simulink model "Aeropendulum_test_simple"  (R2021b)
settings: Solver=VariableStepAuto  StartTime=0.0  StopTime=10.0  RelTol=1e-3
values from neighbouring files (symbols this model uses):
  c = 0.007    [ANM_params.m]    (also in ANM_params_test.m)
  d = 0.25    [ANM_params.m]    (also in ANM_params_test.m)
  g = 9.81    [ANM_params.m]    (also in ANM_params_test.m)
  J = m*l*l    (= 0.0075)    [ANM_params.m]    (also in ANM_params_test.m)
  l = 0.25    [ANM_params.m]    (also in ANM_params_test.m)
  m = 0.120    (= 0.12)    [ANM_params.m]    (also in ANM_params_test.m)
  Rs = 5    [ANM_params.m]
libraries: simulink x1
settings Model: Creator=Marcin  LastModifiedBy=Marcin

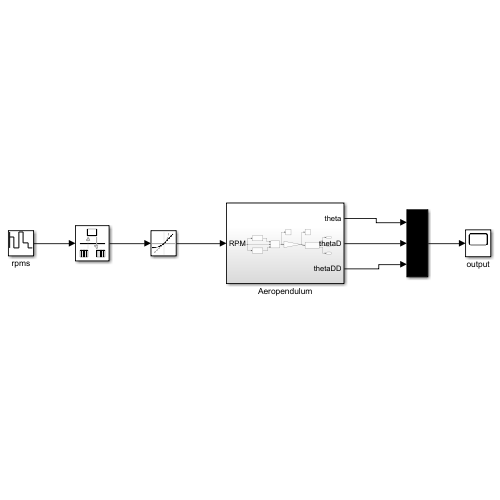
[thumbnail: Simulink's stored preview of the top-level diagram]
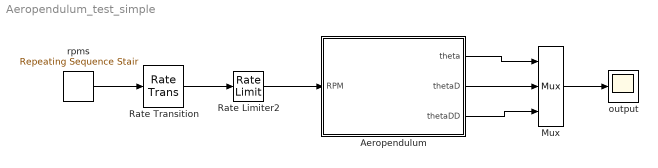
== system Aeropendulum_test_simple ==
  Aeropendulum : Subsystem
  Mux : Mux  Inputs=3
  Rate Limiter2 : RateLimiter  RisingSlewLimit=Rs  FallingSlewLimit=-Rs  SampleTimeMode=inherited
  Rate Transition : RateTransition  InitialCondition=10  OutPortSampleTime=Ts
  output : Scope
  rpms : simulink/Sources/Repeating Sequence Stair  OutValues=input_yref_vector  tsamp=Ts  OutMin=[]  OutMax=[]  OutDataTypeStr=double  OutputDataTypeScalingMode=double  OutDataType=fixdt(0,8)  ConRadixGroup=Best Precision: Vector-wise  OutScaling=2^-12
  wires:
  Rate Transition/1 -> Rate Limiter2/1
  rpms/1 -> Rate Transition/1
  Mux/1 -> output/1
  Aeropendulum/1(theta) -> Mux/1
  Aeropendulum/2(thetaD) -> Mux/2
  Aeropendulum/3(thetaDD) -> Mux/3
  Rate Limiter2/1 -> Aeropendulum/1(RPM)

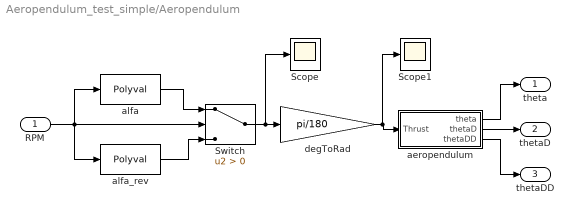
== system Aeropendulum_test_simple/Aeropendulum ==
  RPM : Inport
  Scope : Scope
  Scope1 : Scope
  Switch : Switch  Criteria=u2 > Threshold
  aeropendulum : Subsystem
  alfa : Polyval  Coefs="[3.04986021927422e-06,  -0.00476887717971010 , 2.51670431281220]"
  alfa_rev : Polyval  Coefs="[-5.46944010985214e-06,\t-0.00938361577873603,\t-2.43262552689868]"
  degToRad : Gain  Gain=pi/180
  theta : Outport
  thetaD : Outport  Port=2
  thetaDD : Outport  Port=3
  wires:
  alfa/1 -> Switch/1
  RPM/1 -> alfa_rev/1, alfa/1, Switch/2
  Switch/1 -> Scope/1, degToRad/1
  degToRad/1 -> Scope1/1, aeropendulum/1(Thrust)
  alfa_rev/1 -> Switch/3
  aeropendulum/1(theta) -> theta/1
  aeropendulum/2(thetaD) -> thetaD/1
  aeropendulum/3(thetaDD) -> thetaDD/1

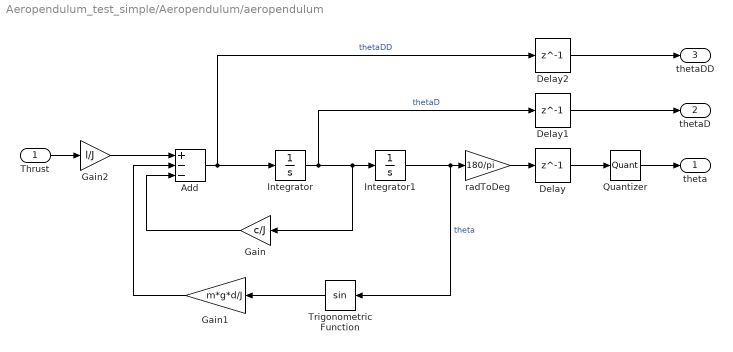
== system Aeropendulum_test_simple/Aeropendulum/aeropendulum ==
  Thrust : Inport
  Add : Sum  Inputs=+--
  Delay : Delay  DelayLength=1  InitialCondition=0
  Delay1 : Delay  DelayLength=1  InitialCondition=0
  Delay2 : Delay  DelayLength=1  InitialCondition=0
  Gain : Gain  Gain=c/J
  Gain1 : Gain  Gain=m*g*d/J
  Gain2 : Gain  Gain=l/J
  Integrator : Integrator
  Integrator1 : Integrator
  Quantizer : Quantizer  QuantizationInterval=0.08791209
  Trigonometric Function : Trigonometry
  radToDeg : Gain  Gain=180/pi
  theta : Outport
  thetaD : Outport  Port=2
  thetaDD : Outport  Port=3
  wires:
  Thrust/1 -> Gain2/1
  Integrator/1 -> Delay1/1, Gain/1, Integrator1/1  "thetaD"
  Integrator1/1 -> Trigonometric Function/1, radToDeg/1  "theta"
  Add/1 -> Delay2/1, Integrator/1  "thetaDD"
  Gain1/1 -> Add/2
  Trigonometric Function/1 -> Gain1/1
  Gain/1 -> Add/3
  Gain2/1 -> Add/1
  radToDeg/1 -> Delay/1
  Delay1/1 -> thetaD/1
  Delay2/1 -> thetaDD/1
  Delay/1 -> Quantizer/1
  Quantizer/1 -> theta/1
